simulink model "APESHI_NO_LOAD"  (R2018a)
settings: Solver=ode45  StartTime=0.0  StopTime=.5  RelTol=1e-3  EnableMultiTasking=on
settings Model: Creator=user  LastModifiedBy=user
settings DataIOCC: LimitDataPoints=on  SaveFormat=Array
settings OptimizationCC: LifeSpan=inf
settings DebuggingCC: SolverPrmCheckMsg=warning  SFUnexpectedBacktrackingDiag=warning  SFNoUnconditionalDefaultTransitionDiag=warning  SFExecutionAtInitializationDiag=none
settings HardwareCC: ProdBitPerPointer=32  ProdBitPerSizeT=32  ProdBitPerPtrDiffT=32  ProdLargestAtomicFloat=None  ProdIntDivRoundTo=Undefined  ProdEndianess=Unspecified  ProdWordSize=32  ProdHWDeviceType=32-bit Generic
settings ModelReferenceCC: PropagateSignalLabelsOutOfModel=off
settings CodeAppCC: StateflowObjectComments=on
settings GRTTargetCC: TargetLangStandard=C89/C90 (ANSI)  GeneratePreprocessorConditionals=Disable all
settings ConfigComp: CovMetricSettings=dw  CovHtmlReporting=on  CovSaveCumulativeToWorkspaceVar=on  CovSaveSingleToWorkspaceVar=on  CovExternalEMLEnable=off  CovSFcnEnable=off

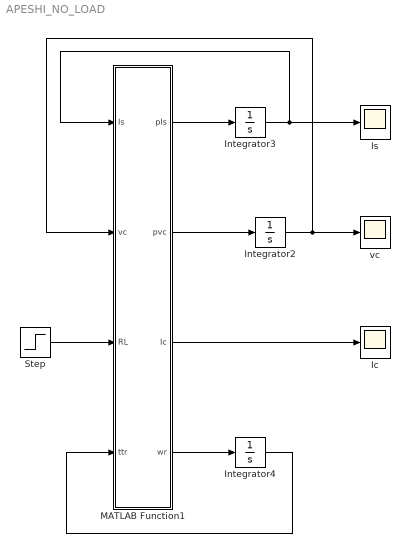
== system APESHI_NO_LOAD ==
  Ic : Scope
  Integrator2 : Integrator  UpperSaturationLimit=.1  LowerSaturationLimit=-.1
  Integrator3 : Integrator  UpperSaturationLimit=.1  LowerSaturationLimit=-.1
  Integrator4 : Integrator  InitialCondition=0.1  LowerSaturationLimit=-0.1
  Is : Scope
  MATLAB Function1 : MATLAB Function  TreatAsAtomicUnit=on
  Step : Step  Time=5  Before=10e9  After=25  SampleTime=0.0001
  vc : Scope
  wires:
  MATLAB Function1/2(pvc) -> Integrator2/1
  Integrator2/1 -> MATLAB Function1/2(vc), vc/1
  MATLAB Function1/4(wr) -> Integrator4/1
  Integrator4/1 -> MATLAB Function1/4(ttr)
  MATLAB Function1/3(Ic) -> Ic/1
  MATLAB Function1/1(pIs) -> Integrator3/1
  Integrator3/1 -> MATLAB Function1/1(Is), Is/1
  Step/1 -> MATLAB Function1/3(RL)

== matlab function APESHI_NO_LOAD/MATLAB Function1 ==
  data: Is input; vc input; pIs output; pvc output; Ic output; wr output; RL input; ttr input
function [pIs,pvc,Ic, wr] =APESHI(Is,vc,RL,ttr)
 
% performance of Single phase permanent magnet synchronous generator on
% Load
% machine parameters
f=50; wr=2*pi*f;xm=0.139;Lmd=0.320;Lmq=0.08; 
L0=(Lmd+Lmq)/2; Ll=(Lmd-Lmq)/2; Ea=2*pi*f*xm*sin(ttr);C=30*10^-6;

Lls=0.067;Rs=27.7;

%single phase self inductance of the machine
Lss=Lls+L0+Ll*cos(2*ttr);
 
% Derivative of the stator current
pIs=inv(Lss)*(Ea-vc+Is*(wr*2*Ll*sin(2*ttr)-Rs));

% % The power factor load
% pf=0.99;
% % the inductive load calculated
% LL=(RL/wr)*sqrt(1/pf)^2-1;
% % the load current
% pIL=(vc-RL*IL)/LL;
% %Load Voltage
% VL=RL*IL+(LL*IL);
% % The power
% Po=vc*Is*pf;
% P=vc*IL*pf;
% Q=vc*IL*(-pf);
% The stator current
Ic=Is;
pvc=(1/C)*Ic;
